simulink subsystem "IMU"  (R2021a)
settings: Solver=VariableStepAuto  StartTime=0.0  StopTime=10.0  RelTol=1e-3
undefined symbols (not defined in the file): biasAcc, biasAng
libraries: simulink x8, dspsrcs4 x2, sharedtransform x1
settings Model: Creator=jmher  LastModifiedBy=jmher

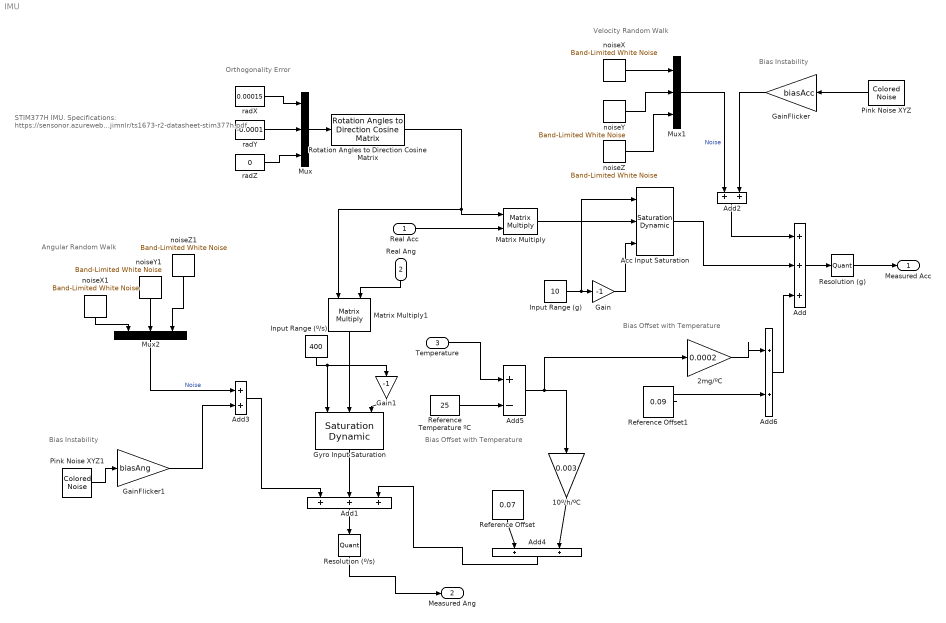
== system IMU ==
  note: Velocity Random Walk
  note: Orthogonality Error
  note: STIM377H IMU.
      |
      | Specifications: https://sensonor.azurewebsites.net/media/qkjimnlr/ts1673-r2-datasheet-stim377h.pdf
  note: Angular Random Walk
  note: Bias Instability
  note: Bias Instability
  note: Bias Offset
      | with Temperature
  note: Bias Offset with Temperature
  Real Acc : Inport  PortDimensions=3
  Real Ang : Inport  Port=2  PortDimensions=3
  Temperature : Inport  Port=3
  10º/h/ºC : Gain  Gain=0.003
  2mg/ºC : Gain  Gain=0.0002
  Acc Input Saturation : simulink/Discontinuities/Saturation Dynamic  OutMin=[]  OutMax=[]  OutDataTypeStr=Inherit: Same as second input  OutDataType=fixdt(1, 16)  OutScaling=2^-10  DoSatur=off
  Add : Sum  Inputs=+|+|+
  Add1 : Sum  Inputs=+|+|+
  Add{2..4,6} (4 alike) : Sum  Inputs=+|+
  Add5 : Sum  Inputs=+|-
  Gain : Gain  Gain=-1
  Gain1 : Gain  Gain=-1
  GainFlicker : Gain  Gain=biasAcc
  GainFlicker1 : Gain  Gain=biasAng
  Gyro Input Saturation : simulink/Discontinuities/Saturation Dynamic  OutMin=[]  OutMax=[]  OutDataTypeStr=Inherit: Same as second input  OutDataType=fixdt(1, 16)  OutScaling=2^-10  DoSatur=off
  Input Range (g) : Constant  Value=10
  Input Range (º/s) : Constant  Value=400
  Matrix Multiply : Product  Multiplication=Matrix(*)
  Matrix Multiply1 : Product  Multiplication=Matrix(*)
  Mux : Mux  Inputs=3
  Mux1 : Mux  Inputs=3
  Mux2 : Mux  Inputs=3
  Pink Noise XYZ : dspsrcs4/Colored Noise  Color=pink  InverseFrequencyPower=biasAcc  BoundedOutput=off  NumChannels=3  OutputDataType=double  SamplesPerFrame=1  SampleTime=0.001  RandomStream=mt19937ar with seed  Seed=67  SimulateUsing=Interpreted execution
      settings: SourceProductBaseCode=DS
  Pink Noise XYZ1 : dspsrcs4/Colored Noise  Color=pink  InverseFrequencyPower=biasAcc  BoundedOutput=off  NumChannels=3  OutputDataType=double  SamplesPerFrame=1  SampleTime=0.001  RandomStream=mt19937ar with seed  Seed=6237  SimulateUsing=Interpreted execution
      settings: SourceProductBaseCode=DS
  Reference Offset : Constant  Value=0.07
  Reference Offset1 : Constant  Value=0.09
  Reference Temperature ºC : Constant  Value=25
  Resolution (g) : Quantizer  QuantizationInterval=1.9e-6  LinearizeAsGain=off
  Resolution (º/s) : Quantizer  QuantizationInterval=0.22  LinearizeAsGain=off
  Rotation Angles to Direction Cosine Matrix : sharedtransform/Rotation Angles to Direction Cosine Matrix  rotationOrder=ZYX  aMode=aMode
      settings: SourceProductBaseCode=AE,PW,DR,MT,UV,VE
  noiseX : simulink/Sources/Band-Limited White Noise  Cov=noiseDensAcc  Ts=0.001  seed=[32323556]
  noiseX1 : simulink/Sources/Band-Limited White Noise  Cov=noiseDensAng  Ts=0.001  seed=[3256]
  noiseY : simulink/Sources/Band-Limited White Noise  Cov=noiseDensAcc  Ts=0.001  seed=[238641]
  noiseY1 : simulink/Sources/Band-Limited White Noise  Cov=noiseDensAng  Ts=0.001  seed=[567380]
  noiseZ : simulink/Sources/Band-Limited White Noise  Cov=noiseDensAcc  Ts=0.001  seed=[23341231]
  noiseZ1 : simulink/Sources/Band-Limited White Noise  Cov=noiseDensAng  Ts=0.001  seed=[234234111]
  radX : Constant  Value=0.00015
  radY : Constant  Value=-0.0001
  radZ : Constant  Value=0
  Measured Acc : Outport  SampleTime=1/40
  Measured Ang : Outport  Port=2  SampleTime=1/40
  wires:
  noiseY/1 -> Mux1/2
  Acc Input Saturation/1 -> Add/2
  Add/1 -> Resolution (g)/1
  noiseZ/1 -> Mux1/3
  noiseX/1 -> Mux1/1
  Gain/1 -> Acc Input Saturation/3
  Gain1/1 -> Gyro Input Saturation/3
  Input Range (g)/1 -> Acc Input Saturation/1, Gain/1
  Resolution (g)/1 -> Measured Acc/1
  Resolution (º/s)/1 -> Measured Ang/1
  radY/1 -> Mux/2
  Mux/1 -> Rotation Angles to Direction Cosine Matrix/1
  radX/1 -> Mux/1
  radZ/1 -> Mux/3
  Rotation Angles to Direction Cosine Matrix/1 -> Matrix Multiply/1, Matrix Multiply1/1
  Real Acc/1 -> Matrix Multiply/2
  Matrix Multiply/1 -> Acc Input Saturation/2
  Gyro Input Saturation/1 -> Add1/2
  Add1/1 -> Resolution (º/s)/1
  noiseY1/1 -> Mux2/2
  noiseZ1/1 -> Mux2/3
  noiseX1/1 -> Mux2/1
  Matrix Multiply1/1 -> Gyro Input Saturation/2
  Mux1/1 -> Add2/1  "Noise"
  Input Range (º/s)/1 -> Gyro Input Saturation/1, Gain1/1
  Mux2/1 -> Add3/1  "Noise"
  Add3/1 -> Add1/1
  Pink Noise XYZ/1 -> GainFlicker/1
  GainFlicker/1 -> Add2/2
  GainFlicker1/1 -> Add3/2
  Pink Noise XYZ1/1 -> GainFlicker1/1
  Real Ang/1 -> Matrix Multiply1/2
  Reference Offset/1 -> Add4/1
  10º/h/ºC/1 -> Add4/2
  Add4/1 -> Add1/3
  Add2/1 -> Add/1
  Reference Offset1/1 -> Add6/2
  Add5/1 -> 2mg/ºC/1, 10º/h/ºC/1
  Add6/1 -> Add/3
  Temperature/1 -> Add5/1
  Reference Temperature ºC/1 -> Add5/2
  2mg/ºC/1 -> Add6/1
